simulink model "ff_test_very_simple"  (R2023b)
settings: Solver=VariableStepAuto  StartTime=0.0  StopTime=10.0  RelTol=1e-3
values from neighbouring files (symbols this model uses):
  K_e = 1    [ff_inv.m]    (also in motor_param.m = 0.00352372567731)
  K_t = 1    [ff_inv.m]    (also in motor_param.m = 0.00352)
  m = 1    [ff_inv.m]    (also in motor_param.m = 0.15)
  R = 1    [ff_inv.m]    (also in motor_param.m = 2.9)
  r = 1    [ff_inv.m]    (also in motor_param.m = 0.012)
settings Model: Creator=under  LastModifiedBy=under

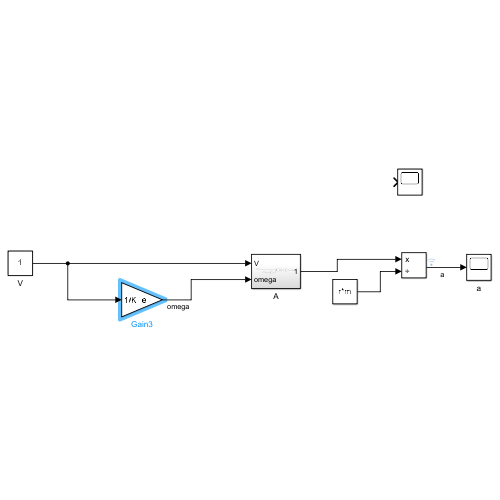
[thumbnail: Simulink's stored preview of the top-level diagram]
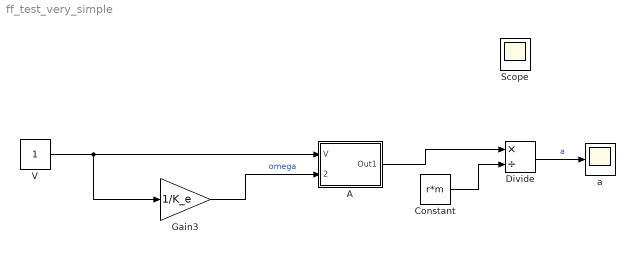
== system ff_test_very_simple ==
  A : Subsystem
  Constant : Constant  Value=r*m
  Divide : Product  Inputs=*/
  Gain3 : Gain  Gain=1/K_e
  Scope : Scope
  V : Constant
  a : Scope
  wires:
  Divide/1 -> a/1  "a"
  V/1 -> Gain3/1, A/1(V)
  Gain3/1 -> A/2(omega)  "omega"
  Constant/1 -> Divide/2
  A/1(Out1) -> Divide/1

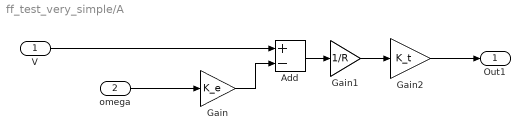
== system ff_test_very_simple/A ==
  V : Inport
  omega : Inport  Port=2
  Add : Sum  Inputs=+-
  Gain : Gain  Gain=K_e
  Gain1 : Gain  Gain=1/R
  Gain2 : Gain  Gain=K_t
  Out1 : Outport
  wires:
  Gain2/1 -> Out1/1
  Gain1/1 -> Gain2/1
  Add/1 -> Gain1/1
  Gain/1 -> Add/2
  omega/1 -> Gain/1
  V/1 -> Add/1
